simulink model "mass_spring2"  (Simulink 8.0)
settings: Solver=ode45  StartTime=0.0  StopTime=10.0  RelTol=1e-3
settings Model: Creator=Tran Minh Luan  LastModifiedBy=Tran Minh Luan

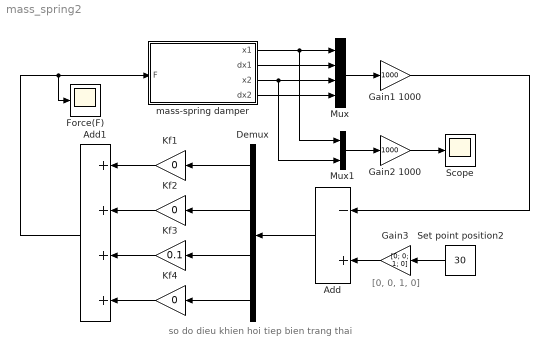
== system mass_spring2 ==
  note: so do dieu khien hoi tiep bien trang thai
  note: [0, 0, 1, 0]
  Add : Sum  Inputs=-+
  Add1 : Sum  Inputs=++++
  Demux : Demux
  Force(F) : Scope
  Gain1 1000 : Gain  Gain=1000
  Gain2 1000 : Gain  Gain=1000
  Gain3 : Gain  Gain=[0; 0; 1; 0]
  Kf1 : Gain  Gain=0
  Kf2 : Gain  Gain=0
  Kf3 : Gain  Gain=0.1
  Kf4 : Gain  Gain=0
  Mux : Mux
  Mux1 : Mux  Inputs=2
  Scope : Scope
  Set point position2 : Constant  Value=30
  mass-spring damper : Subsystem
  wires:
  mass-spring damper/1(x1) -> Mux1/1, Mux/1
  mass-spring damper/2(dx1) -> Mux/2
  mass-spring damper/3(x2) -> Mux1/2, Mux/3
  mass-spring damper/4(dx2) -> Mux/4
  Mux/1 -> Gain1 1000/1
  Gain3/1 -> Add/2
  Set point position2/1 -> Gain3/1
  Gain1 1000/1 -> Add/1
  Mux1/1 -> Gain2 1000/1
  Gain2 1000/1 -> Scope/1
  Add/1 -> Demux/1
  Demux/1 -> Kf1/1
  Demux/2 -> Kf2/1
  Demux/3 -> Kf3/1
  Demux/4 -> Kf4/1
  Kf1/1 -> Add1/1
  Kf2/1 -> Add1/2
  Kf3/1 -> Add1/3
  Kf4/1 -> Add1/4
  Add1/1 -> Force(F)/1, mass-spring damper/1(F)

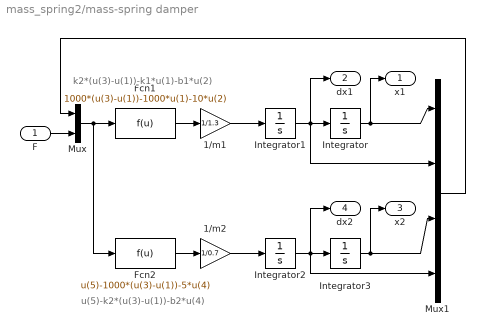
== system mass_spring2/mass-spring damper ==
  note: u(5)-k2*(u(3)-u(1))-b2*u(4)
  note: k2*(u(3)-u(1))-k1*u(1)-b1*u(2)
  F : Inport
  1/m1 : Gain  Gain=1/1.3
  1/m2 : Gain  Gain=1/0.7
  "Fcn1 " : Fcn  Expr=1000*(u(3)-u(1))-1000*u(1)-10*u(2)
  "Fcn2 " : Fcn  Expr=u(5)-1000*(u(3)-u(1))-5*u(4)
  Integrator{,1..3} (4 alike) : Integrator
  Mux : Mux  Inputs=2
  Mux1 : Mux
  x1 : Outport
  dx1 : Outport  Port=2
  x2 : Outport  Port=3
  dx2 : Outport  Port=4
  wires:
  F/1 -> Mux/2
  1/m1/1 -> Integrator1/1
  Integrator1/1 -> Integrator/1, dx1/1, Mux1/2
  Integrator/1 -> Mux1/1, x1/1
  Integrator3/1 -> Mux1/3, x2/1
  Integrator2/1 -> Integrator3/1, dx2/1, Mux1/4
  1/m2/1 -> Integrator2/1
  Mux1/1 -> Mux/1
  Mux/1 -> "Fcn2 "/1, "Fcn1 "/1
  "Fcn1 "/1 -> 1/m1/1
  "Fcn2 "/1 -> 1/m2/1
